simulink model "linearized_doubletank"  (R2024b)
settings: Solver=VariableStepAuto  StartTime=0.0  StopTime=500  RelTol=1e-3
values from neighbouring files (symbols this model uses):
  K = 4    [TankSystem.m]    (also in matlabGraphsForLabA.mat = [0.0280520906769 0.0679241172515])
  T = 35    [TankSystem.m]    (also in matlabGraphsForLabA.mat)
libraries: simulink x2
settings Model: Creator=William  LastModifiedBy=William

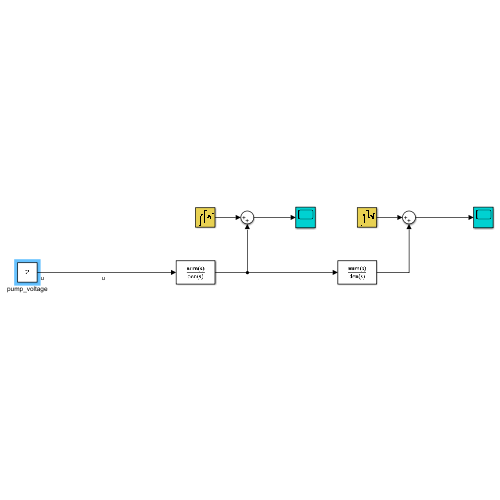
[thumbnail: Simulink's stored preview of the top-level diagram]
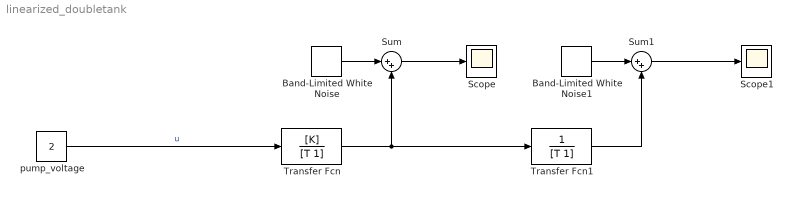
== system linearized_doubletank ==
  Band-Limited White Noise : simulink/Sources/Band-Limited White Noise  Cov=[2e-6]  Ts=0.1  seed=[23341]
  Band-Limited White Noise1 : simulink/Sources/Band-Limited White Noise  Cov=[2e-6]  Ts=0.1  seed=[23341]
  Scope : Scope
  Scope1 : Scope
  Sum : Sum  Inputs=|++
  Sum1 : Sum  Inputs=|++
  Transfer Fcn : TransferFcn  Numerator=[K]  Denominator=[T 1]
  Transfer Fcn1 : TransferFcn  Denominator=[T 1]
  pump_voltage : Constant  Value=2
  wires:
  pump_voltage/1 -> Transfer Fcn/1  "u"
  Transfer Fcn/1 -> Sum/2, Transfer Fcn1/1
  Sum/1 -> Scope/1
  Band-Limited White Noise/1 -> Sum/1
  Sum1/1 -> Scope1/1
  Transfer Fcn1/1 -> Sum1/2
  Band-Limited White Noise1/1 -> Sum1/1
